simulink model "Example1"  (R2023a)
settings: Solver=VariableStepAuto  StartTime=0.0  StopTime=10.0  RelTol=1e-3
settings Model: Creator=The MathWorks, Inc.  LastModifiedBy=admin
settings SolverCC: MaxZcPerStep=1
settings DebuggingCC: UnconnectedInputMsg=warning  UnconnectedOutputMsg=warning  UnconnectedLineMsg=warning
settings ModelReferenceCC: EnableRefExpFcnMdlSchedulingChecks=on
settings RTWCC: DLArmComputeVersion=19.05

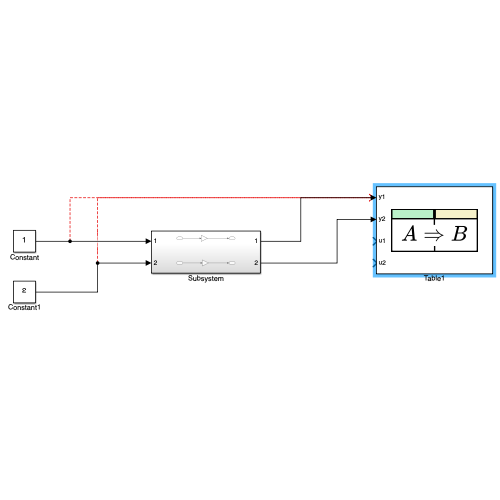
[thumbnail: Simulink's stored preview of the top-level diagram]
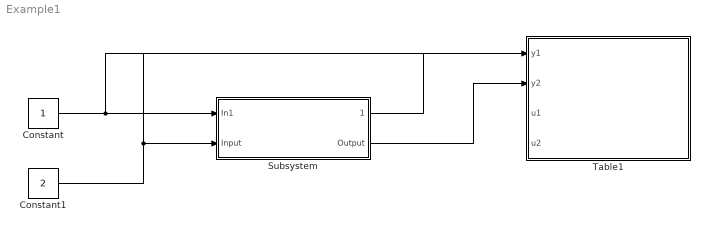
== system Example1 ==
  Constant : Constant
  Constant1 : Constant  Value=2
  Subsystem : Subsystem
  Table1 : Requirements Table  TreatAsAtomicUnit=on
  wires:
  Subsystem/2(Output) -> Table1/2(y2)
  Constant/1 -> Subsystem/1(In1)
  Constant1/1 -> Subsystem/2(Input)
  Subsystem/1(1) -> Table1/1(y1)

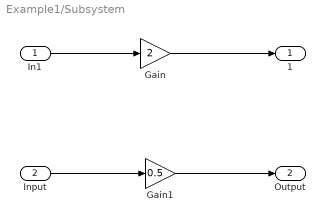
== system Example1/Subsystem ==
  In1 : Inport
  Input : Inport  Port=2
  Gain : Gain  Gain=2
  Gain1 : Gain  Gain=0.5
  1 : Outport
  Output : Outport  Port=2
  wires:
  Gain/1 -> 1/1
  In1/1 -> Gain/1
  Input/1 -> Gain1/1
  Gain1/1 -> Output/1

== stateflow chart Example1/Table1 ==
  (default) -> (junction 1073742791)
  (junction 1073742791) -> (junction 1073742792) : {
      | % SF_REQ_REV_07
      | }
  (junction 1073742792) -> (junction 1073742794) : {
      | % HEADER_ASSIGNMENTS
      |
      | }
  (junction 1073742794) -> (junction 1073742796) : {
      | % START_A_4
      | }
  (junction 1073742796) -> (junction 1073742798) : {
      | }
  (junction 1073742798) -> (junction 1073742800)
  (junction 1073742800) -> (junction 1073742802) : {
      | }
  (junction 1073742802) -> (junction 1073742804) : {
      | % END_A_4
      | }
  (junction 1073742804) -> (junction 1073742806) : {
      | % START_R_7
      | }
  (junction 1073742806) -> (junction 1073742808) : {
      | }
  (junction 1073742808) -> (junction 1073742810)
  (junction 1073742810) -> (junction 1073742812) [order 1] : [(u1==prev(u1)+1)]
  (junction 1073742810) -> (junction 1073742818) [order 2]
  (junction 1073742812) -> (junction 1073742814) : {
      | reqtable_postcondition((y1 == prev(y1)+2), 'R:1');
      |
      |
      | }
  (junction 1073742814) -> (junction 1073742816) : {
      | }
  (junction 1073742816) -> (junction 1073742818)
  (junction 1073742818) -> (junction 1073742820)
  (junction 1073742820) -> (junction 1073742822) : {
      | % END_R_7
      | }
  (junction 1073742822) -> (junction 1073742824) : {
      | % START_R_1
      | }
  (junction 1073742824) -> (junction 1073742826) : {
      | }
  (junction 1073742826) -> (junction 1073742828)
  (junction 1073742828) -> (junction 1073742830) [order 1] : [(u2 > 2)]
  (junction 1073742828) -> (junction 1073742836) [order 2]
  (junction 1073742830) -> (junction 1073742832) : {
      | reqtable_postcondition((y2 > 5), 'R:2');
      |
      |
      | }
  (junction 1073742832) -> (junction 1073742834) : {
      | }
  (junction 1073742834) -> (junction 1073742836)
  (junction 1073742836) -> (junction 1073742838)
  (junction 1073742838) -> (junction 1073742840) : {
      | % END_R_1
      | }
  data: y1 input double; y2 input double; u1 input double; data local; u2 input double
